simulink model "BEML_EMU_TestBench_6Car"  (R2019b)
settings: Solver=VariableStepAuto  StartTime=0.0  StopTime=inf  RelTol=1e-3
PreLoadFcn:
  | set_up_test_modelCB_6Car;
undefined symbols (not defined in the file): Common, IOControls, MaxVehicles, MotionBaseControllerInput, VehicleInputs, VehicleType, Z_CfgVehBus
libraries: TestBenchLib x583, simulink x6
(part 3 of 3)

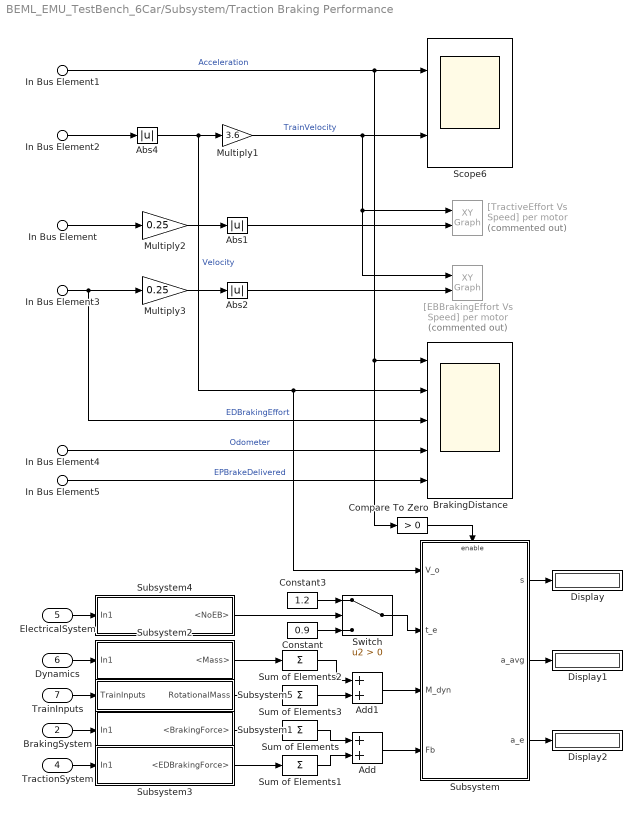
== system BEML_EMU_TestBench_6Car/Subsystem/Traction Braking Performance ==
  In Bus Element1 : Inport  PortName=DynamicsLastCab  Element=Inertia.Acceleration
  In Bus Element2 : Inport  PortName=DynamicsLastCab  Element=Inertia.Velocity
  BrakingSystem : Inport  Port=2
  In Bus Element : Inport  Port=3  PortName=TCMSOut  Element=Display.TractionBraking.TractiveEffort
  In Bus Element3 : Inport  Port=3  PortName=TCMSOut  Element=Display.TractionBraking.VehicleEDBrakingEffortAchieved
  In Bus Element5 : Inport  Port=3  PortName=TCMSOut  Element=Display.TractionBraking.EPBrakeDelivered
  In Bus Element4 : Inport  Port=3  PortName=TCMSOut  Element=Display.ElectricalSystem.Odometer
  TractionSystem : Inport  Port=4
  ElectricalSystem : Inport  Port=5
  Dynamics : Inport  Port=6
  TrainInputs : Inport  Port=7
  Abs1 : Abs
  Abs2 : Abs
  Abs4 : Abs
  Add : Sum
  Add1 : Sum
  BrakingDistance : Scope  NumInputPorts=5
  Compare To Zero : simulink/Logic and Bit Operations/Compare To Zero  relop=>  OutDataTypeStr=boolean
  Constant : Constant  Value=0.9
  Constant3 : Constant  Value=1.2
  Display : Display
  Display1 : Display
  Display2 : Display
  Multiply1 : Gain  Gain=3.6
  Multiply2 : Gain  Gain=0.25
  Multiply3 : Gain  Gain=0.25
  Scope6 : Scope  NumInputPorts=2
  Subsystem : Subsystem
  Subsystem1 : Subsystem
  Subsystem2 : Subsystem
  Subsystem3 : Subsystem
  Subsystem4 : Subsystem
  Subsystem5 : Subsystem
  Sum of Elements{,1..3} (4 alike) : Sum  Inputs=+
  Switch : Switch  Criteria=u2 > Threshold
  "[EBBrakingEffort Vs Speed] per motor" : simulink/Sinks/XY Graph  Commented=on  xmin=0  xmax=100  ymin=0  ymax=25000  st=-1
  "[TractiveEffort Vs Speed] per motor" : simulink/Sinks/XY Graph  Commented=on  xmin=0  xmax=100  ymin=0  ymax=35000  st=-1
  wires:
  In Bus Element2/1 -> Abs4/1
  Multiply1/1 -> "[EBBrakingEffort Vs Speed] per motor"/1, "[TractiveEffort Vs Speed] per motor"/1, Scope6/2  "TrainVelocity"
  In Bus Element/1 -> Multiply2/1
  Abs1/1 -> "[TractiveEffort Vs Speed] per motor"/2
  Abs2/1 -> "[EBBrakingEffort Vs Speed] per motor"/2
  Multiply2/1 -> Abs1/1
  In Bus Element3/1 -> BrakingDistance/3, Multiply3/1  "EDBrakingEffort"
  Multiply3/1 -> Abs2/1
  In Bus Element1/1 -> Compare To Zero/1, BrakingDistance/1, Scope6/1  "Acceleration"
  Abs4/1 -> Subsystem/1(V_o), BrakingDistance/2, Multiply1/1  "Velocity"
  In Bus Element4/1 -> BrakingDistance/4  "Odometer"
  In Bus Element5/1 -> BrakingDistance/5  "EPBrakeDelivered"
  Constant/1 -> Switch/3
  Subsystem/1(s) -> Display/1
  Subsystem/2(a_avg) -> Display1/1
  Subsystem/3(a_e) -> Display2/1
  Compare To Zero/1 -> Subsystem/Enable
  BrakingSystem/1 -> Subsystem1/1(In1)
  Subsystem1/1(<BrakingForce>) -> Sum of Elements/1
  Dynamics/1 -> Subsystem2/1(In1)
  Subsystem2/1(<Mass>) -> Sum of Elements2/1
  Sum of Elements/1 -> Add/1
  TractionSystem/1 -> Subsystem3/1(In1)
  Subsystem3/1(<EDBrakingForce>) -> Sum of Elements1/1
  Add/1 -> Subsystem/4(Fb)
  Sum of Elements1/1 -> Add/2
  ElectricalSystem/1 -> Subsystem4/1(In1)
  Subsystem4/1(<NoEB>) -> Switch/2
  Switch/1 -> Subsystem/2(t_e)
  Constant3/1 -> Switch/1
  Add1/1 -> Subsystem/3(M_dyn)
  Subsystem5/1(RotationalMass) -> Sum of Elements3/1
  Sum of Elements2/1 -> Add1/1
  TrainInputs/1 -> Subsystem5/1(TrainInputs)
  Sum of Elements3/1 -> Add1/2

== system BEML_EMU_TestBench_6Car/Subsystem/Train Config Creator For Testing ==
  Constant : Constant  Value=Z_CfgVehBus  VectorParams1D=off  OutDataTypeStr=Bus: BD_SimIntegration_Cfg_Vehicle
  OldConfigWayViaBlocks : Subsystem  Commented=on
  VehicleConfig : Outport  VectorParamsAs1DForOutWhenUnconnected=off
  wires:
  Constant/1 -> VehicleConfig/1

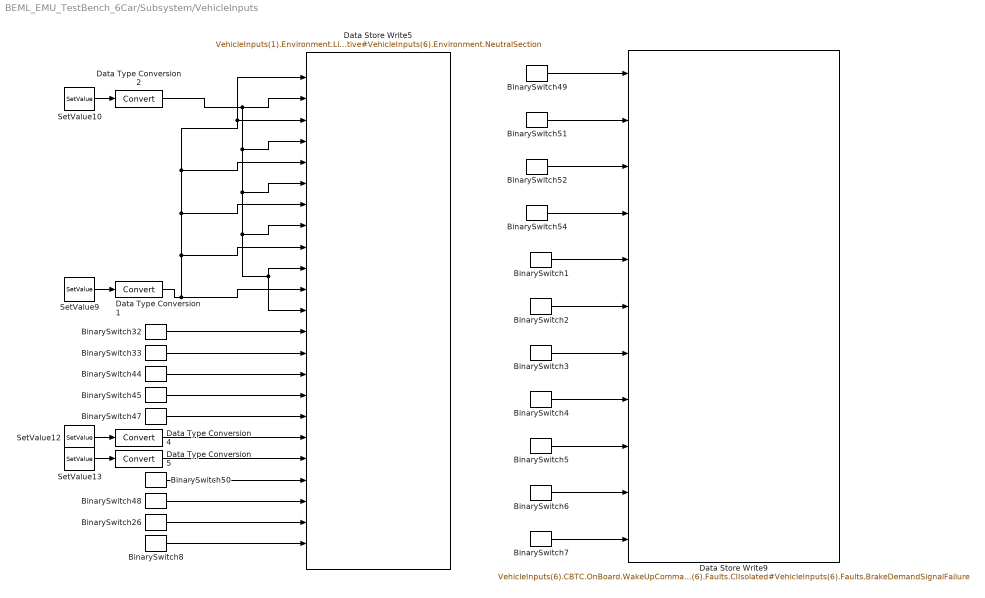
== system BEML_EMU_TestBench_6Car/Subsystem/VehicleInputs ==
  BinarySwitch{1..8,26,44..45,48..52,54} (17 alike) : TestBenchLib/BinarySwitch  value=0  init_value=0  block_colour=[0 1 0]  WorkspaceVarName=0
      settings: SourceProductName=Sydac Utilities
  BinarySwitch32 : TestBenchLib/BinarySwitch  value=1  init_value=1  block_colour=[0 1 0]  WorkspaceVarName=0
      settings: SourceProductName=Sydac Utilities
  BinarySwitch33 : TestBenchLib/BinarySwitch  value=1  init_value=1  block_colour=[0 1 0]  WorkspaceVarName=0
      settings: SourceProductName=Sydac Utilities
  BinarySwitch47 : TestBenchLib/BinarySwitch  value=1  init_value=1  block_colour=[0 1 0]  WorkspaceVarName=0
      settings: SourceProductName=Sydac Utilities
  Data Store Write5 : DataStoreWrite  Priority=1  DataStoreName=VehicleInputs  DataStoreElements=VehicleInputs(1).Environment.LineVoltage#VehicleInputs(1).Environment.OverheadLinePresent#VehicleInputs(2).Environment.LineVoltage#VehicleInputs(2).Environment.OverheadLinePresent#VehicleInputs(3).Environment.LineVoltage#VehicleInputs(3).Environment.OverheadLinePresent#VehicleInputs(4).Environment.LineVoltage#VehicleInputs(4).Environment.OverheadLinePresent#VehicleInputs(5).Environment.LineVoltage#VehicleInputs(5).Environment.OverheadLinePresent#VehicleInputs(6).Environment.LineVoltage#VehicleInputs(6).Environment.OverheadLinePresent#VehicleInputs(6).CBTC.OnBoard.NoServiceBrakeOrder#VehicleInputs(6).CBTC.OnBoard.NoEmergencyBrakeOrder#VehicleInputs(2).Environment.NeutralSection#VehicleInputs(5).Environment.NeutralSection#VehicleInputs(6).CBTC.OnBoard.ImmobilisationState#VehicleInputs(6).CBTC.OnBoard.ATOPermittedSpeed#VehicleInputs(6).CBTC.OnBoard.ATOPermittedDistance#VehicleInputs(6).CBTC.OnBoard.ATOStartIndicator#VehicleInputs(6).CBTC.OnBoard.ATOState#VehicleInputs(6).CBTC.OnBoard.UTOModeActive#VehicleInputs(6).Environment.NeutralSection
  Data Store Write9 : DataStoreWrite  Priority=1  DataStoreName=VehicleInputs  DataStoreElements=VehicleInputs(6).CBTC.OnBoard.WakeUpCommand#VehicleInputs(6).CBTC.OnBoard.ATCCabActivation#VehicleInputs(1).CBTC.OnBoard.ATCCabActivation#VehicleInputs(6).CBTC.OnBoard.TractionForward#VehicleInputs(6).Faults.OHLHighVoltageLevel3#VehicleInputs(6).Faults.OHLLowVoltageLevel2#VehicleInputs(3).Faults.BICContactorActivationFault#VehicleInputs(6).Faults.EmergencyDoorMechanicalUnlocked#VehicleInputs(6).Faults.CIFailure#VehicleInputs(6).Faults.CIIsolated#VehicleInputs(6).Faults.BrakeDemandSignalFailure
  Data Type Conversion{1..2,4..5} (4 alike) : DataTypeConversion
  SetValue10 : TestBenchLib/SetValue  value=1  init_value=1  WorkspaceVarName=0
      settings: SourceProductName=Sydac Utilities
  SetValue12 : TestBenchLib/SetValue  value=5  init_value=5  WorkspaceVarName=0
      settings: SourceProductName=Sydac Utilities
  SetValue13 : TestBenchLib/SetValue  value=500  init_value=500  WorkspaceVarName=0
      settings: SourceProductName=Sydac Utilities
  SetValue9 : TestBenchLib/SetValue  value=25000  init_value=25000  WorkspaceVarName=0
      settings: SourceProductName=Sydac Utilities
  wires:
  SetValue9/1 -> Data Type Conversion1/1
  Data Type Conversion1/1 -> Data Store Write5/11, Data Store Write5/9, Data Store Write5/7, Data Store Write5/5, Data Store Write5/1, Data Store Write5/3
  Data Type Conversion2/1 -> Data Store Write5/4, Data Store Write5/6, Data Store Write5/8, Data Store Write5/10, Data Store Write5/12, Data Store Write5/2
  SetValue10/1 -> Data Type Conversion2/1
  SetValue13/1 -> Data Type Conversion5/1
  SetValue12/1 -> Data Type Conversion4/1
  BinarySwitch49/1 -> Data Store Write9/1
  BinarySwitch51/1 -> Data Store Write9/2
  BinarySwitch54/1 -> Data Store Write9/4
  BinarySwitch52/1 -> Data Store Write9/3
  BinarySwitch32/1 -> Data Store Write5/13
  BinarySwitch33/1 -> Data Store Write5/14
  BinarySwitch44/1 -> Data Store Write5/15
  BinarySwitch45/1 -> Data Store Write5/16
  BinarySwitch47/1 -> Data Store Write5/17
  BinarySwitch50/1 -> Data Store Write5/20
  BinarySwitch48/1 -> Data Store Write5/21
  BinarySwitch26/1 -> Data Store Write5/22
  Data Type Conversion4/1 -> Data Store Write5/18
  Data Type Conversion5/1 -> Data Store Write5/19
  BinarySwitch2/1 -> Data Store Write9/6
  BinarySwitch1/1 -> Data Store Write9/5
  BinarySwitch3/1 -> Data Store Write9/7
  BinarySwitch4/1 -> Data Store Write9/8
  BinarySwitch5/1 -> Data Store Write9/9
  BinarySwitch6/1 -> Data Store Write9/10
  BinarySwitch7/1 -> Data Store Write9/11
  BinarySwitch8/1 -> Data Store Write5/23

== system BEML_EMU_TestBench_6Car/Subsystem/ZeroSpeedFromATC ==
  note: ZeroSpeed from CBTC?
  In1 : Inport
  In2 : Inport  Port=2
  Abs : Abs
  Abs1 : Abs
  BinarySwitch53 : TestBenchLib/BinarySwitch  value=1  init_value=1  block_colour=[0 1 0]  WorkspaceVarName=0
      settings: SourceProductName=Sydac Utilities
  Bus Selector : BusSelector  OutputSignals=Inertia.Velocity
  Bus Selector1 : BusSelector  OutputSignals=TCMS.CabActive
  Bus Selector2 : BusSelector  OutputSignals=Inertia.Velocity
  Bus Selector3 : BusSelector  OutputSignals=TCMS.CabActive
  Compare To Constant : simulink/Logic and Bit Operations/Compare To Constant  relop=<=  const=0.05  OutDataTypeStr=boolean
  Compare To Constant1 : simulink/Logic and Bit Operations/Compare To Constant  relop=<=  const=0.05  OutDataTypeStr=boolean
  DMC1 : Selector  InputPortWidth=MaxVehicles  IndexOptions=Index vector (dialog)  Indices=1  OutputSizes=1
  DMC1. : Selector  InputPortWidth=MaxVehicles  IndexOptions=Index vector (dialog)  Indices=1  OutputSizes=1
  DMC2 : Selector  InputPortWidth=MaxVehicles  IndexOptions=Index vector (dialog)  Indices=6  OutputSizes=1
  DMC2. : Selector  InputPortWidth=MaxVehicles  IndexOptions=Index vector (dialog)  Indices=6  OutputSizes=1
  Data Store Write9 : DataStoreWrite  Priority=1  DataStoreName=VehicleInputs  DataStoreElements=VehicleInputs(1).CBTC.OnBoard.ZeroSpeed#VehicleInputs(6).CBTC.OnBoard.ZeroSpeed
  Data Type Conversion : DataTypeConversion
  Data Type Conversion1 : DataTypeConversion
  Logical Operator : Logic  Inputs=3  AllPortsSameDT=off  OutDataTypeStr=boolean
  Logical Operator1 : Logic  Inputs=3  AllPortsSameDT=off  OutDataTypeStr=boolean
  wires:
  In1/1 -> DMC2/1, DMC1/1
  DMC2/1 -> Bus Selector/1
  In2/1 -> DMC1./1, DMC2./1
  DMC2./1 -> Bus Selector1/1
  DMC1/1 -> Bus Selector2/1
  DMC1./1 -> Bus Selector3/1
  Bus Selector1/1 -> Logical Operator/3  "<CabActive>"
  Bus Selector2/1 -> Abs/1  "<Velocity>"
  Bus Selector3/1 -> Logical Operator1/3  "<CabActive>"
  Bus Selector/1 -> Abs1/1  "<Velocity>"
  Logical Operator/1 -> Data Type Conversion1/1
  Logical Operator1/1 -> Data Type Conversion/1
  Data Type Conversion/1 -> Data Store Write9/1
  Data Type Conversion1/1 -> Data Store Write9/2
  Abs/1 -> Compare To Constant/1
  Compare To Constant/1 -> Logical Operator1/2
  Abs1/1 -> Compare To Constant1/1
  Compare To Constant1/1 -> Logical Operator/2
  BinarySwitch53/1 -> Logical Operator/1, Logical Operator1/1

== system BEML_EMU_TestBench_6Car/Subsystem/DoorSystemTest/Subsystem ==
  <Doors> : Inport  Partition=on  PartitionDimension=1  PartitionWidth=1  PartitionOffset=0
  Bus Selector1 : BusSelector  OutputSignals=OutputControlStates.DoorPosition,OutputControlStates.DoorOutsideLamp,OutputControlStates.DoorInsideLamp
  For Each : ForEach  DisableCoverage=on
  <DoorPosition> : Outport  ConcatenationDimension=1
  DoorOutsideLamp : Outport  Port=2  ConcatenationDimension=1
  DoorInsideLamp : Outport  Port=3  ConcatenationDimension=1
  wires:
  <Doors>/1 -> Bus Selector1/1
  Bus Selector1/1 -> <DoorPosition>/1  "<DoorPosition>"
  Bus Selector1/2 -> DoorOutsideLamp/1  "<DoorOutsideLamp>"
  Bus Selector1/3 -> DoorInsideLamp/1  "<DoorInsideLamp>"

== system BEML_EMU_TestBench_6Car/Subsystem/DoorSystemTest/Subsystem1 ==
  <Doors> : Inport  Partition=on  PartitionDimension=1  PartitionWidth=1  PartitionOffset=0
  Bus Selector1 : BusSelector  OutputSignals=OutputControlStates.DoorPosition,OutputControlStates.DoorOutsideLamp,OutputControlStates.DoorInsideLamp
  For Each : ForEach  DisableCoverage=on
  <DoorPosition> : Outport  ConcatenationDimension=1
  DoorOutsideLamp : Outport  Port=2  ConcatenationDimension=1
  DoorInsideLamp : Outport  Port=3  ConcatenationDimension=1
  wires:
  <Doors>/1 -> Bus Selector1/1
  Bus Selector1/1 -> <DoorPosition>/1  "<DoorPosition>"
  Bus Selector1/2 -> DoorOutsideLamp/1  "<DoorOutsideLamp>"
  Bus Selector1/3 -> DoorInsideLamp/1  "<DoorInsideLamp>"

== system BEML_EMU_TestBench_6Car/Subsystem/DoorSystemTest/Subsystem2 ==
  <Doors> : Inport  Partition=on  PartitionDimension=1  PartitionWidth=1  PartitionOffset=0
  Bus Selector1 : BusSelector  OutputSignals=OutputControlStates.DoorPosition,OutputControlStates.DoorOutsideLamp,OutputControlStates.DoorInsideLamp
  For Each : ForEach  DisableCoverage=on
  <DoorPosition> : Outport  ConcatenationDimension=1
  DoorOutsideLamp : Outport  Port=2  ConcatenationDimension=1
  DoorInsideLamp : Outport  Port=3  ConcatenationDimension=1
  wires:
  <Doors>/1 -> Bus Selector1/1
  Bus Selector1/1 -> <DoorPosition>/1  "<DoorPosition>"
  Bus Selector1/2 -> DoorOutsideLamp/1  "<DoorOutsideLamp>"
  Bus Selector1/3 -> DoorInsideLamp/1  "<DoorInsideLamp>"

== system BEML_EMU_TestBench_6Car/Subsystem/DoorSystemTest/Subsystem3 ==
  <Doors> : Inport  Partition=on  PartitionDimension=1  PartitionWidth=1  PartitionOffset=0
  Bus Selector1 : BusSelector  OutputSignals=OutputControlStates.DoorPosition,OutputControlStates.DoorOutsideLamp,OutputControlStates.DoorInsideLamp
  For Each : ForEach  DisableCoverage=on
  <DoorPosition> : Outport  ConcatenationDimension=1
  DoorOutsideLamp : Outport  Port=2  ConcatenationDimension=1
  DoorInsideLamp : Outport  Port=3  ConcatenationDimension=1
  wires:
  <Doors>/1 -> Bus Selector1/1
  Bus Selector1/1 -> <DoorPosition>/1  "<DoorPosition>"
  Bus Selector1/2 -> DoorOutsideLamp/1  "<DoorOutsideLamp>"
  Bus Selector1/3 -> DoorInsideLamp/1  "<DoorInsideLamp>"

== system BEML_EMU_TestBench_6Car/Subsystem/Traction Braking Performance/Subsystem ==
  V_o : Inport
  t_e : Inport  Port=2
  M_dyn : Inport  Port=3
  Fb : Inport  Port=4
  Enable : EnablePort
  Add : Sum
  Divide : Product  Inputs=*/
  Divide1 : Product  Inputs=*/
  Divide2 : Product  Inputs=*/
  Gain : Gain  Gain=2
  Gain1 : Gain  Gain=2
  Product : Product
  Square : Math  Operator=square  SignedPower=off  SaturateOnIntegerOverflow=on
  s : Outport
  a_avg : Outport  Port=2
  a_e : Outport  Port=3
  wires:
  Add/1 -> Gain1/1, s/1  "s"
  Divide/1 -> Add/2
  Gain/1 -> Divide/2
  V_o/1 -> Square/1, Product/1
  Divide1/1 -> a_e/1, Gain/1  "a_e"
  Square/1 -> Divide2/1, Divide/1
  Product/1 -> Add/1
  t_e/1 -> Product/2
  M_dyn/1 -> Divide1/2
  Gain1/1 -> Divide2/2
  Divide2/1 -> a_avg/1
  Fb/1 -> Divide1/1

== system BEML_EMU_TestBench_6Car/Subsystem/Traction Braking Performance/Subsystem1 ==
  In1 : Inport  Partition=on  PartitionDimension=1  PartitionWidth=1  PartitionOffset=0
  Bus Selector : BusSelector  OutputSignals=Axle
  For Each : ForEach  DisableCoverage=on
  Subsystem2 : Subsystem
  Sum of Elements : Sum  Inputs=+
  <BrakingForce> : Outport  ConcatenationDimension=1
  wires:
  In1/1 -> Bus Selector/1
  Bus Selector/1 -> Subsystem2/1(In1)  "<Axle>"
  Subsystem2/1(<BrakingForce>) -> Sum of Elements/1
  Sum of Elements/1 -> <BrakingForce>/1

== system BEML_EMU_TestBench_6Car/Subsystem/Traction Braking Performance/Subsystem2 ==
  In1 : Inport  Partition=on  PartitionDimension=1  PartitionWidth=1  PartitionOffset=0
  Bus Selector : BusSelector  OutputSignals=Inertia
  For Each : ForEach  DisableCoverage=on
  Subsystem2 : Subsystem
  Sum of Elements : Sum  Inputs=+
  <Mass> : Outport  ConcatenationDimension=1
  wires:
  Sum of Elements/1 -> <Mass>/1
  Subsystem2/1(<Mass>) -> Sum of Elements/1
  Bus Selector/1 -> Subsystem2/1(In1)  "<Inertia>"
  In1/1 -> Bus Selector/1

== system BEML_EMU_TestBench_6Car/Subsystem/Traction Braking Performance/Subsystem3 ==
  In1 : Inport  Partition=on  PartitionDimension=1  PartitionWidth=1  PartitionOffset=0
  Bus Selector : BusSelector  OutputSignals=Dynamics
  For Each : ForEach  DisableCoverage=on
  Subsystem2 : Subsystem
  Sum of Elements : Sum  Inputs=+
  <EDBrakingForce> : Outport  ConcatenationDimension=1
  wires:
  Sum of Elements/1 -> <EDBrakingForce>/1
  Subsystem2/1(<BrakingForce>) -> Sum of Elements/1
  Bus Selector/1 -> Subsystem2/1(In1)  "<Dynamics>"
  In1/1 -> Bus Selector/1

== system BEML_EMU_TestBench_6Car/Subsystem/Traction Braking Performance/Subsystem4 ==
  In1 : Inport  Partition=on  PartitionDimension=1  PartitionWidth=1  PartitionOffset=0
  Bus Selector : BusSelector  OutputSignals=Braking
  For Each : ForEach  DisableCoverage=on
  OR : Logic  Operator=OR  Inputs=1  AllPortsSameDT=off  OutDataTypeStr=boolean
  Subsystem2 : Subsystem
  <NoEB> : Outport  ConcatenationDimension=1
  wires:
  In1/1 -> Bus Selector/1
  Bus Selector/1 -> Subsystem2/1(In1)  "<Braking>"
  Subsystem2/1(<NoEB>) -> OR/1
  OR/1 -> <NoEB>/1

== system BEML_EMU_TestBench_6Car/Subsystem/Traction Braking Performance/Subsystem5 ==
  TrainInputs : Inport  Partition=on  PartitionDimension=1  PartitionWidth=1  PartitionOffset=0
  Bus Selector : BusSelector  OutputSignals=Electrical
  For Each : ForEach  DisableCoverage=on
  Subsystem : Subsystem
  RotationalMass : Outport  ConcatenationDimension=1
  wires:
  TrainInputs/1 -> Bus Selector/1
  Bus Selector/1 -> Subsystem/1(<Electrical>)  "<Electrical>"
  Subsystem/1(Out1) -> RotationalMass/1

== system BEML_EMU_TestBench_6Car/Subsystem/Train Config Creator For Testing/OldConfigWayViaBlocks ==
  Assignment{,1..3} (4 alike) : Assignment  DiagnosticForDimensions=Warning  IndexOptions=Starting index (dialog)  Indices=1  OutputSizes=1
  Full Lenght  Orientation2 : Constant  Value=[1 1 2 2 1 1 2 2 1 1 2 2 1 1 2 2]
  Full Lenght Unit 4 Car Class1 : Constant  Value=[851 853 852 854 851 853 852 854]
  Full Lenght Unit 4 Car Class2 : Constant  Value=[851 853 852 854 851 853 852 854 851 853 852 854 851 853 852 854]
  Full Lenght Unit 4 Car Class4 : Constant  Value=[851 853 852 854]
  Full Lenght Unit 4 Car Class5 : Constant  Value=[851 853 852 854 851 853 852 854 851 853 852 854]
  Full Lenght Unit 4 Car Mass 1 : Constant  Value=[39008 36850 36450 31170 39008 36850 36450 31170]
  Full Lenght Unit 4 Car Mass 3 : Constant  Value=[39008 36850 36450 31170 39008 36850 36450 31170 39008 36850 36450 31170 39008 36850 36450 31170]
  Full Lenght Unit 4 Car Mass 4 : Constant  Value=[39008 36850 36450 31170]
  Full Lenght Unit 4 Car Mass 5 : Constant  Value=[39008 36850 36450 31170 39008 36850 36450 31170 39008 36850 36450 31170]
  Full Lenght Unit 4 Car Orientation1 : Constant  Value=[1 1 2 2 1 1 2 2]
  Full Lenght Unit 4 Car Orientation4 : Constant  Value=[1 1 2 2 ]
  Full Lenght Unit 4 Car Orientation5 : Constant  Value=[1 1 2 2 1 1 2 2 1 1 2 2 ]
  Full Lenght Unit 4 cars1 : Constant  Value=[VehicleType.Motor VehicleType.Motor VehicleType.Motor VehicleType.Motor VehicleType.Motor VehicleType.Motor VehicleType.Motor VehicleType.Motor VehicleType.Motor VehicleType.Motor VehicleType.Motor VehicleType.Motor VehicleType.Motor VehicleType.Motor VehicleType.Motor VehicleType.Motor]
  Full Lenght Unit 4 cars3 : Constant  Value=[VehicleType.Motor VehicleType.Motor VehicleType.Motor VehicleType.Motor ]
  Full Lenght Unit 4 cars4 : Constant  Value="[VehicleType.Motor VehicleType.Motor VehicleType.Motor VehicleType.Motor VehicleType.Motor VehicleType.Motor VehicleType.Motor VehicleType.Motor VehicleType.Motor VehicleType.Motor VehicleType.Motor VehicleType.Motor  VehicleType.Motor VehicleType.Motor VehicleType.Motor VehicleType.Motor ]"
  Full Length Unit IDs1 : Constant  Value=[1 1 1 1 2 2 2 2]
  Full Length Unit IDs4 : Constant  Value=[1 1 1 1]
  Max Vehicle1 : Constant  Value=zeros(MaxVehicles, 1, 'VehicleType')
  Max Vehicle5 : Constant  Value=zeros(MaxVehicles, 1, 'VehicleType')
  Max Vehicle6 : Constant  Value=zeros(MaxVehicles, 1)
  Max Vehicle7 : Constant  Value=zeros(MaxVehicles, 1)
  Subsystem : Subsystem
  CommonVehicleConfig : Outport  VectorParamsAs1DForOutWhenUnconnected=off
  wires:
  Full Lenght Unit 4 cars4/1 -> Assignment/2
  Max Vehicle1/1 -> Assignment/1
  Full Lenght Unit 4 Car Class2/1 -> Assignment1/2
  Full Lenght  Orientation2/1 -> Assignment2/2
  Assignment/1 -> Subsystem/1(Type)
  Assignment1/1 -> Subsystem/2(Class)
  Assignment2/1 -> Subsystem/3(Orientation)
  Subsystem/1(Out1) -> CommonVehicleConfig/1
  Max Vehicle7/1 -> Assignment3/1, Assignment2/1, Assignment1/1
  Full Lenght Unit 4 Car Mass 3/1 -> Assignment3/2
  Assignment3/1 -> Subsystem/4(TareMass)
  Full Lenght Unit 4 Car Class1/1 -> ?
  Max Vehicle6/1 -> ?
  Full Length Unit IDs1/1 -> ?
  Full Length Unit IDs4/1 -> ?
  Full Lenght Unit 4 Car Orientation4/1 -> ?
  Full Lenght Unit 4 Car Orientation1/1 -> ?
  Full Lenght Unit 4 Car Mass 5/1 -> ?
  Full Lenght Unit 4 Car Mass 1/1 -> ?
  Full Lenght Unit 4 Car Class5/1 -> ?
  Full Lenght Unit 4 Car Class4/1 -> ?
  Full Lenght Unit 4 Car Orientation5/1 -> ?
  Full Lenght Unit 4 cars1/1 -> ?

== system BEML_EMU_TestBench_6Car/Subsystem/Traction Braking Performance/Subsystem1/Subsystem2 ==
  In1 : Inport  Partition=on  PartitionDimension=1  PartitionWidth=1  PartitionOffset=0
  Bus Selector : BusSelector  OutputSignals=BrakingForce
  For Each : ForEach  DisableCoverage=on
  <BrakingForce> : Outport  ConcatenationDimension=1
  wires:
  Bus Selector/1 -> <BrakingForce>/1  "<BrakingForce>"
  In1/1 -> Bus Selector/1

== system BEML_EMU_TestBench_6Car/Subsystem/Traction Braking Performance/Subsystem2/Subsystem2 ==
  In1 : Inport  Partition=on  PartitionDimension=1  PartitionWidth=1  PartitionOffset=0
  Bus Selector : BusSelector  OutputSignals=Mass
  For Each : ForEach  DisableCoverage=on
  <Mass> : Outport  ConcatenationDimension=1
  wires:
  In1/1 -> Bus Selector/1
  Bus Selector/1 -> <Mass>/1  "<Mass>"

== system BEML_EMU_TestBench_6Car/Subsystem/Traction Braking Performance/Subsystem3/Subsystem2 ==
  In1 : Inport  Partition=on  PartitionDimension=1  PartitionWidth=1  PartitionOffset=0
  Bus Selector : BusSelector  OutputSignals=BrakingForce
  For Each : ForEach  DisableCoverage=on
  <BrakingForce> : Outport  ConcatenationDimension=1
  wires:
  In1/1 -> Bus Selector/1
  Bus Selector/1 -> <BrakingForce>/1  "<BrakingForce>"

== system BEML_EMU_TestBench_6Car/Subsystem/Traction Braking Performance/Subsystem4/Subsystem2 ==
  In1 : Inport  Partition=on  PartitionDimension=1  PartitionWidth=1  PartitionOffset=0
  Bus Selector : BusSelector  OutputSignals=NoEB
  For Each : ForEach  DisableCoverage=on
  <NoEB> : Outport  ConcatenationDimension=1
  wires:
  Bus Selector/1 -> <NoEB>/1  "<NoEB>"
  In1/1 -> Bus Selector/1

== system BEML_EMU_TestBench_6Car/Subsystem/Traction Braking Performance/Subsystem5/Subsystem ==
  <Electrical> : Inport  Partition=on  PartitionDimension=1  PartitionWidth=1  PartitionOffset=0
  Bus Selector1 : BusSelector  OutputSignals=IsT1,IsT2,IsT3
  For Each : ForEach  DisableCoverage=on
  Gain : Gain  Gain=2
  M_rot : Constant  Value=2100
  OR : Logic  Operator=OR  Inputs=3  AllPortsSameDT=off  OutDataTypeStr=boolean
  Switch : Switch  Criteria=u2 > Threshold
  Out1 : Outport  ConcatenationDimension=1
  wires:
  Gain/1 -> Switch/3
  <Electrical>/1 -> Bus Selector1/1
  OR/1 -> Switch/2  "IsTCar"
  M_rot/1 -> Gain/1, Switch/1
  Bus Selector1/2 -> OR/2  "<IsT2>"
  Bus Selector1/3 -> OR/3  "<IsT3>"
  Bus Selector1/1 -> OR/1  "<IsT1>"
  Switch/1 -> Out1/1

== system BEML_EMU_TestBench_6Car/Subsystem/Train Config Creator For Testing/OldConfigWayViaBlocks/Subsystem ==
  note: Will need to update this Wheel Diameters
  Type : Inport  Partition=on  PartitionDimension=1  PartitionWidth=1  PartitionOffset=0
  Class : Inport  Port=2  Partition=on  PartitionDimension=1  PartitionWidth=1  PartitionOffset=0
  Orientation : Inport  Port=3  Partition=on  PartitionDimension=1  PartitionWidth=1  PartitionOffset=0
  TareMass : Inport  Port=4  Partition=on  PartitionDimension=1  PartitionWidth=1  PartitionOffset=0
  Bus Assignment : BusAssignment  AssignedSignals=Common.Enabled,Common.Type,Common.Class,Common.Orientation,Common.Length,Common.Height,Common.Width,Common.TareMass,Common.GrossMass,Common.LoadingMass,Common.WheelDiameter
  Compare To Constant : simulink/Logic and Bit Operations/Compare To Constant  relop=~=  const=VehicleType.NoVehicleType  OutDataTypeStr=boolean
  Constant : Constant  Value=0  OutDataTypeStr=Bus: BD_TrainModel_Cfg_Vehicle
  For Each : ForEach  DisableCoverage=on
  GrossMass : Constant  Value=55000
  Height : Constant  Value=3.849
  Length : Constant  Value=26
  LoadingMass : Constant  Value=0
  WheelDiameter : Constant  Value=0.83
  Width : Constant  Value=2.74
  Out1 : Outport  ConcatenationDimension=1  VectorParamsAs1DForOutWhenUnconnected=off
  wires:
  Type/1 -> Bus Assignment/3, Compare To Constant/1  "Type"
  Width/1 -> Bus Assignment/8  "Width"
  Height/1 -> Bus Assignment/7  "Height"
  TareMass/1 -> Bus Assignment/9  "TareMass"
  GrossMass/1 -> Bus Assignment/10  "GrossMass"
  Constant/1 -> Bus Assignment/1
  Bus Assignment/1 -> Out1/1
  LoadingMass/1 -> Bus Assignment/11  "LoadingMass"
  Orientation/1 -> Bus Assignment/5  "Orientation"
  Class/1 -> Bus Assignment/4  "Class"
  Length/1 -> Bus Assignment/6  "Length"
  Compare To Constant/1 -> Bus Assignment/2  "Enabled"
  WheelDiameter/1 -> Bus Assignment/12
